simulink model "sensorFusionWithControlTB66StatePos"  (R2024a)
settings: Solver=FixedStepAuto  StartTime=0.0  StopTime=inf  FixedStep=controlRate  RelTol=1e-3
InitFcn:
  | modelParamsDD = Simulink.data.dictionary.open('modelConfigData.sldd');
  | sectModel = getSection(modelParamsDD,'Design Data');
  | controlRateTemp = getValue(getEntry(sectModel,'controlRate'));
  | 
  | measRate = controlRateTemp;
  | angleEstRate = measRate;
  | stateEstRate = measRate;
  | 
  | 
  | % Complementary filter
  | fc = 5; %Hz
  | tau = 1/(2*pi*fc);
  | alpha = tau/(tau+controlRateTemp);
  | 
  | % Control params
  | tiltSetPoint = 1; % degree
  | 
  | % Tilt angle PID
  | Tw = 1;
  | Kp = 17;
  | Ki = 4; %
  | Kd = 0;
  | 
  | % Velocity angle PID
  | Tw_vel = 1;
  | Kp_vel = 17;
  | Ki_vel = 4;
  | Kd_vel = 0;
  | 
  | % Position angle PID
  | targetPosition = 0.1;
  | Tw_pos = 1;
  | Kp_pos = 17;
  | Ki_pos = 4;
  | Kd_pos = 0;
  | 
  | clear controlRateTemp
  | 
  | motorParamsDD = Simulink.data.dictionary.open('motorParametersData.sldd');
  | robotParamsDD = Simulink.data.dictionary.open('robotModelData.sldd');
  | controlParamsDD = Simulink.data.dictionary.open('controlVariablesData.sldd');
  | sectMotor = getSection(motorParamsDD,'Design Data');
  | sectRobot = getSection(robotParamsDD,'Design Data');
  | sectControl = getSection(controlParamsDD,'Design Data');
  | 
  | % Physical Parameters
  | M = getValue(getEntry(sectRobot,'massOfCart'));    % mass of cart
  | m = getValue(getEntry(sectRobot,'massOfPendulum'));    % mass of pendulum
  | L = getValue(getEntry(sectRobot,'lengthToPendulumCenterOfMass'));    % length to pendulum center of mass
  | g = 9.81;   % gravity
  | I = getValue(getEntry(sectRobot,'inertiaOfPendulum'));  % inertia of pendulum
  | r = getValue(getEntry(sectRobot,'wheelRadius'));   % 5 cm wheel radius
  | 
  | % Servo motor state: i, omega
  | Rm = getValue(getEntry(sectMotor,'armatureResistance')); % motor resistance
  | Lm = getValue(getEntry(sectMotor,'armatureInductance')); % motor coil inductance
  | Km = getValue(getEntry(sectMotor,'motorTorqueConstantKm')); % motor torque constant
  | Kb = getValue(getEntry(sectMotor,'backEMFConstantKb')); % motor electrical consant
  | Kf = getValue(getEntry(sectMotor,'viscousFriction')); % viscous friction
  | J = getValue(getEntry(sectMotor,'motorInertia'));  % inertia of rotor
  | 
  | Q_aug_lqr = getValue(getEntry(sectControl,'Q_aug_lqr'));
  | R_aug_lqr = getValue(getEntry(sectControl,'R_aug_lqr'));
  | 
  | % States are x, dx/dt, phi, dphi/dt
  | % Outputs are x position and tilt angle
  | 
  | % Linearized state-space model of inverted pendulum
  | I_tot = m*L^2+I;
  | p = m^2*L^2 - I_tot*(M+m);
  | A_pend = [0 1 0 0;
  |           0 0 (m^2 * g * L^2)/p 0;
  |           0 0 0 1;
  |           0 0 -(M+m)/(m*L)*m^2*L^2*g/p 0];
  | 
  | B_pend = [0; -I_tot/p; 0; 1/(m*L)*(1+(M+m)*I_tot/p)];
  | 
  | C_pend = [1 0 0 0;
  |           0 0 1 0];
  | D_pend = zeros(2,1);
  | 
  | % Discretize System - for the augmented system
  | sysd = c2d(ss(A_pend, B_pend, C_pend, D_pend), measRate);
  | Ad_pend = single(sysd.A);
  | Bd_pend = single(sysd.B);
  | Cd_pend = single(sysd.C);
  | Dd_pend = single(sysd.D);
  | 
  | % State-space model: output is torque = Km * i
  | A_motor = [-Rm/L,   -Kb/Lm;
  |             Km/J, -Kf/J];
  | B_motor = [1/Lm;
  |            0];
  | C_motor = [Km*(1/r), 0];  % Output is torque = Km * i
  | D_motor = 0;
  | 
  | % Augment System: Force = torque / r
  | % States are x, dx/dt, phi, dphi/dt, i, w
  | % Outputs are x position and tilt angle
  | 
  | A_aug = [A_pend, B_pend*C_motor;
  |          zeros(2,4), A_motor];
  | 
  | B_aug = [B_pend*D_motor; B_motor];
  | 
  | C_aug = [C_pend, D_pend*C_motor];
  | n_aug = size(A_aug,1);
  | 
  | 
  | % Discretize System - for the augmented system
  | sysd = c2d(ss(A_aug, B_aug, C_aug, 0), measRate);
  | Ad_aug = single(sysd.A);
  | Bd_aug = single(sysd.B);
  | Cd_aug = single(sysd.C);
  | 
  | clear J Kt M m l g I r Q_lqr_temp R_lqr_temp dt
  | clear Rm Lm Km Kb Kf J
  | clear motorParamsDD robotParamsDD controlParamsDD modelParamsDD sectMotor sectRobot sectControl sectModel sysd
  | 
  | % LQR Controller matrices (moved here from SLDD to be tuned)
  | Q_aug_lqr_temp = [0.1 0 0 0 0 0;0 0.1 0 0 0 0;0 0 10 0 0 0;0 0 0 50 0 0;0 0 0 0 0.1 0;0 0 0 0 0 0.1];
  | R_aug_lqr_temp = 30;
  | 
  | % LQR Controller - for the augmented system
  | [K_aug_lqr, ~, ~] = dlqr(Ad_aug, Bd_aug, Q_aug_lqr, R_aug_lqr);
  | K_aug_lqr = single(K_aug_lqr);
undefined symbols (not defined in the file or in its folder): accelToUnit, controlRate, gyroToUnit, MaxMotorVoltage, posControlRate
libraries: stm32blockslib x2, stm32f7xxblockslib x2, stm32f4xxblockslib x1
settings Model: DataDictionary=globalData.sldd  VariantConfigurationObject=RobotVariantConfig  STM32="{\"PWMOutput\":[{\"ID\":\"sensorFusionWithControlTB66State:205\"},{\"ID\":\"sensorFusionWithControlTB66State:189\"},{\"ID\":\"sensorFusionWithControlTB66StatePos:2012\"},{\"ID\":\"sensorFusionWithControlTB66StatePos:2013\"}],\"DigitalPortWrite\":[{\"ID\":\"sensorFusionWithControlTB66State:1189\"},{\"ID\":\"sensorFusionWithControlTB66State:1225:7\"},{\"ID\":\"sensorFusionWithControlTB66State:1225:8\"},{\"ID\":\"sensorFusionWithControlTB66State:1225:9\"},{\"ID\":\"sensorFusionWithControlTB66State:1225:10\"},{\"ID\":\"sensorFusionWithControlTB66StatePos:1992\"},{\"ID\":\"sensorFusionWithControlTB66StatePos:2051:7\"},{\"ID\":\"sensorFusionWithControlTB66StatePos:2051:8\"},{\"ID\":\"sensorFusionWithControlTB66StatePos:2051:9\"},{\"ID\":\"sensorFusionWithControlTB66StatePos:2051:10\"}],\"EncoderBlock\":[{\"ID\":\"sensorFusionWithControlTB66State:1254\"},{\"ID\":\"sensorFusionWithControlTB66State:1257\"},{\"ID\":\"sensorFusionWithControlTB66StatePos:1993\"},{\"ID\":\"sensorFusionWithControlTB66StatePos:1994\"}],\"I2CControllerRead\":[{\"ID\":\"sensorFusionWithControlTB66State:1237:7\"},{\"ID\":\"sensorFusionWithControlTB66State:1237:18\"},{\"ID\":\"sensorFusionWithControlTB66State:1237:19\"},{\"ID\":\"sensorFusionWithControlTB66State:1237:20\"},{\"ID\":\"sensorFusionWithControlTB66State:1238:7\"},{\"ID\":\"sensorFusionWithControlTB66State:1238:15\"},{\"ID\":\"sensorFusionWithControlTB66State:1238:16\"},{\"ID\":\"sensorFusionWithControlTB66State:1238:17\"},{\"ID\":\"sensorFusionWithControlTB66StatePos:1237:18\"},{\"ID\":\"sensorFusionWithControlTB66StatePos:1237:19\"},{\"ID\":\"sensorFusionWithControlTB66StatePos:1237:20\"},{\"ID\":\"sensorFusionWithControlTB66StatePos:1238:7\"},{\"ID\":\"sensorFusionWithControlTB66StatePos:1238:15\"},{\"ID\":\"sensorFusionWithControlTB66StatePos:1238:16\"},{\"ID\":\"sensorFusionWithControlTB66StatePos:1238:17\"},{\"ID\":\"sensorFusionWithControlTB66StatePos:2053:7\"},{\"ID\":\"sensorFusionWithControlTB66StatePos:2053:18\"},{\"ID\":\"sensorFusionWithControlTB66StatePos:2053:19\"},{\"ID\":\"sensorFusionWithControlTB66StatePos:2053:20\"},{\"ID\":\"sensorFusionWithControlTB66StatePos:2054:7\"},{\"ID\":\"sensorFusionWithControlTB66StatePos:2054:15\"},{\"ID\":\"sensorFusionWithControlTB66StatePos:2054:16\"},{\"ID\":\"sensorFusionWithControlTB66StatePos:2054:17\"}],\"I2CControllerWrite\":[{\"ID\":\"sensorFusionWithControlTB66State:1237:21\"},{\"ID\":\"sensorFusionWithControlTB66State:1237:22\"},{\"ID\":\"sensorFusionWithControlTB66State:1237:23\"},{\"ID\":\"sensorFusionWithControlTB66State:1238:18\"},{\"ID\":\"sensorFusionWithControlTB66State:1238:19\"},{\"ID\":\"sensorFusionWithControlTB66State:1238:20\"},{\"ID\":\"sensorFusionWithControlTB66StatePos:1237:21\"},{\"ID\":\"sensorFusionWithControlTB66StatePos:1237:22\"},{\"ID\":\"sensorFusionWithControlTB66StatePos:1237:23\"},{\"ID\":\"sensorFusionWithControlTB66StatePos:1238:18\"},{\"ID\":\"sensorFusionWithControlTB66StatePos:1238:19\"},{\"ID\":\"sensorFusionWithControlTB66StatePos:1238:20\"},{\"ID\":\"sensorFusionWithControlTB66StatePos:2053:21\"},{\"ID\":\"sensorFusionWithControlTB66StatePos:2053:22\"},{\"ID\":\"sensorFusionWithControlTB66StatePos:2053:23\"},{\"ID\":\"sensorFusionWithControlTB66StatePos:2054:18\"},{\"ID\":\"sensorFusionWithControlTB66StatePos:2054:19\"},{\"ID\":\"sensorFusionWithControlTB66StatePos:2054:20\"}]}"  SimulationMode=external  Creator=Peter  LastModifiedBy=Peter
settings OptimizationCC: OptimizeBlockIOStorage=off  BufferReuse=off  ReuseModelBlockBuffer=off  GlobalBufferReuse=off  ExpressionFolding=off  EnableMemcpy=off  PassReuseOutputArgsAs=Individual arguments  LocalBlockOutputs=off  ZeroExternalMemoryAtStartup=off  ZeroInternalMemoryAtStartup=off  MaxStackSize=64  OptimizeDataStoreBuffers=off  BusAssignmentInplaceUpdate=off  OptimizationLevel=level0  OptimizationCustomize=off  EfficientTunableParamExpr=on
settings DebuggingCC: ParameterTunabilityLossMsg=error
settings HardwareCC: ProdBitPerPointer=32  ProdBitPerSizeT=32  ProdBitPerPtrDiffT=32  ProdLargestAtomicInteger=Long  ProdLargestAtomicFloat=Double  ProdWordSize=32  ProdLongLongMode=on  ProdHWDeviceType=ARM Compatible->ARM Cortex-M
settings SFSimCC: MATLABDynamicMemAlloc=off
settings RTWCC: Description=Embedded Coder  SystemTargetFile=ert.tlc  HardwareBoard=STM32F7xx Based (Single precision FPU)  GenCodeOnly=on  TemplateMakefile=ert_default_tmf  Toolchain=GNU Tools for ARM Embedded Processors
settings CodeAppCC: GenerateComments=off  IgnoreCustomStorageClasses=off  OperatorAnnotations=on  SimulinkDataObjDesc=on  SFDataObjDesc=on  SimulinkBlockComments=off
settings ERTTargetCC: TargetLangStandard=C99 (ISO)  CodeReplacementLibrary=ARM Cortex-M  SupportComplex=off  ExtMode=on  ExtModeTransport=3  ExtModeStaticAlloc=on  ExtModeStaticAllocSize=2048  ExtModeMexFile=ext_xcp  ExtModeMexArgs=1 'COM11' 115200  ExtModeIntrfLevel=Level2 - Open

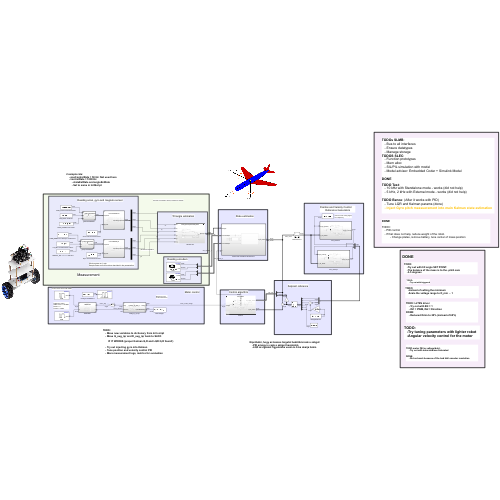
[thumbnail: Simulink's stored preview of the top-level diagram]
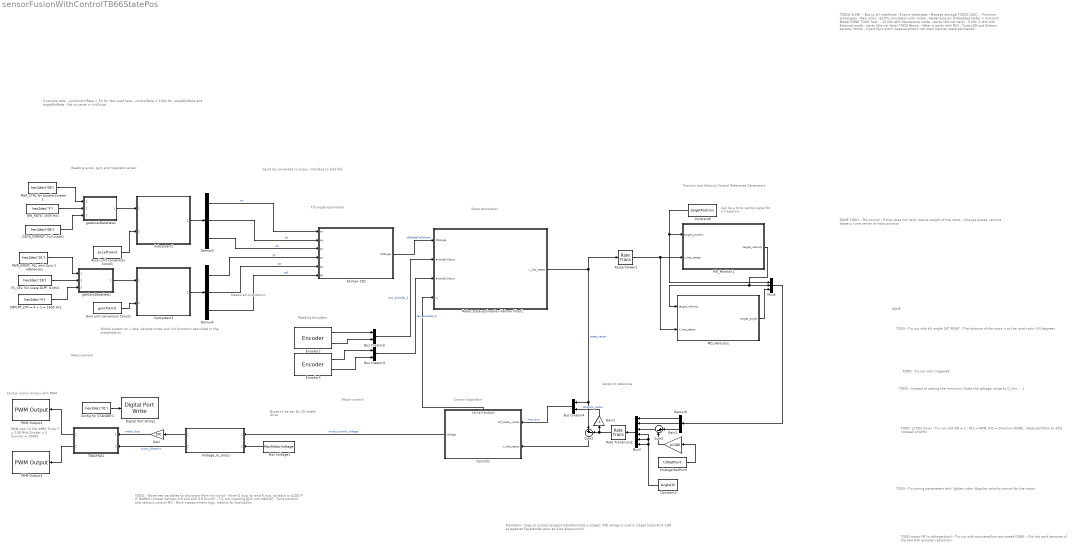
== system sensorFusionWithControlTB66StatePos ==
  note: Control algorithm
  note: Control motor dirvers with PWM
  note: TODO:
      | -Try out with tilt angle SET POINT.
      | -The balance of the mass is to the -pitch axis
      | -3-5 degrees
  note: TODO motor FB (w voltage/duty)
      | - Try out with saturated/non saturated
      |
      | DONE:
      | - Did not work because of the bad Hall encoder resolution
  note: Reading accel, gyro and megneto sensor
  note: Measured orientation
  note: 2 sample rate:
      | - posControlRate = 50 Hz: Not used here
      | - controlRate = 1000 Hz
      | - stateEstRate and angleEstRate
      | - Set to same in InitScript
  note: PWM with 10 kHz
      | APB2 Timer f = 108 MHz
      | Divider = 0
      | Counter = 10800
  note: Measurement
  note: Motor control
  note: Whole system on 1 rate.
      | Sample times and init functions described in the presentation.
  note: Buses to be set
      | for 2D wheel drive
  note: State estimation
  note: Setpoint reference
  note: Tilt angle estimation
  note: TODO:
      | -Try tuning parameters with lighter robot
      | -Angular velocity control for the motor
  note: Reading encoders
  note: Could be converted to buses, interface to sldd file
  note: TODO:
      | -Try out with triggered
  note: TODO: L279N driver
      | - Try out with EN = 1
      | - IN1 = PWM, IN2 = Direction
      | DONE:
      | - Reduced Dmin to 20% (instead of 60%)
  note: DONE
  note: TODO:
      | -Instead of setting the minimum
      | -Scale the voltage range to D_min ... 1
  note: DONE
      |
      | TODO:
      | - PID control
      | - If that does not help, reduce weight of the robot.
      | - Change plates, remove battery, tune center of mass position
  note: TODOs SLMB :
      | - Bus to all interfaces
      | - Ensure datatypes
      | - Manage storage
      | TODOS SLEC :
      | - Function prototypes
      | - Mem alloc
      | - SIL/PIL simulation with model
      | - Model advisor: Embedded Coder + Simulink Model
      |
      | DONE
      |
      | TODO Test :
      | - 10 kHz with Standalone mode - works (did not help)
      | - 5 kHz, 2 kHz with External mode - works (did not help)
      |
      | TODO Bence : (After it works with PID)
      | - Tune LQR and Kalman params (done)
      | - Inject Gyro pitch measuerement into main Kalman state estimation
  note: TODO:
      | - Move new variables to dictionary from Init script
      | - Move Q_aug_lqr and R_aug_lqr back to SLDD
      |
      | IF IT WORKS (proper Kalman Q,R and LQR Q,R found!)
      |
      | - Try out injecting gyro into Kalman
      | - Tune position and velocity control PID
      | - More measurement logs, metrics for evaluation
  note: Can be a time varing signal
      | for a trajectory
  note: Kipróbálni, hogy az összes targetot bekötöm/csak a szöget:
      | -PID amúgy is csak a szöget használná
      | -LQR az egészet figyelembe veszi és 0-ba akarja húzni.
  note: Position and Velocity Control
      | Reference Generators
  Accel unit conversion Const1 : Constant  Value=accelToUnit  OutDataTypeStr=single
  BW_RATE: 1600 Hz1 : Constant  Value=hex2dec('F')  OutDataTypeStr=uint8
  Bus Creator2 : BusCreator  Inputs=2
  Bus Creator3 : BusCreator  Inputs=2
  Bus Creator4 : BusCreator  Inputs=2
  Config for STANDBY1 : Constant  Value=hex2dec('01')  OutDataTypeStr=uint8
  Constant2 : Constant  Value=single(0)
  Constant6 : Constant  Value=targetPosition  OutDataTypeStr=single
  Control1 : Subsystem  Variant=on  VariantChoicesEnumeration=controlEnumState  VariantControlVariable=controlAlgStateCtrl  VariantControl=Subsystem2  VariantActivationTime=inherit from Simulink.VariantControl
      settings: PortSchema="{\"entries\":[{\"content\":{\"sides\":[{\"content\":{\"connectorIds\":[\"In1\",\"In2\"]},\"type\":\"ConnectorPlacement.EquallySpacedRectSide\",\"uuid\":\"f699f757-4844-4aff-9ceb-41d5b2044f89\"},{\"content\":{\"connectorIds\":[\"Out1\"],\"side\":\"RIGHT\"},\"type\":\"ConnectorPlacement.EquallySpacedRectSide\",\"uuid\":\"5d4ff76b-5e14-4a3a-b7d6-9f05c394657c\"},{\"content\":{\"connectorIds\":[\"Out2\"],\"side\":\"TOP\"},\"type\":\"ConnectorPlacement.EquallySpacedRectSide\",\"uuid\":\"774b8687-b42a-4b88-b210-7c8eb4b61568\"}]},\"type\":\"ConnectorPlacement.EquallySpacedConnector\",\"uuid\":\"f6913896-c1bf-44b7-bb24-894f4bed7d15\"}],\"packageUris\":[\"http://schema.mathworks.com/mf0/Connector/R2020b\"],\"version\":\"1.0\"}"
  DATA_FORMAT: Full scale1 : Constant  Value=hex2dec('0B')  OutDataTypeStr=uint8
  Demux3 : Demux  Outputs=3
  Demux4 : Demux  Outputs=3
  Demux6 : Demux  Outputs=3
  Digital Port Write1 : stm32f4xxblockslib/Digital Port Write  PortName=GPIOF  PinNumber=[13]  ReadOperation=off  IOAsArray=off  EnableSimPort=off  hoistedMaskSrc=ECSoC/ECSimCodegen/Digital Port Write
      settings: LibrarySourceBlock=stm32f7xxblockslib/Digital Port Write
  Encoder2 : stm32blockslib/Encoder  TimerModule=TIM1  EnableResetInput=off  OutputDirection=on  SampleTime=angleEstRate
      settings: LibrarySourceBlock=stm32f7xxblockslib/Encoder
  Encoder3 : stm32blockslib/Encoder  TimerModule=TIM3  EnableResetInput=off  OutputDirection=on  SampleTime=angleEstRate
      settings: LibrarySourceBlock=stm32f7xxblockslib/Encoder
  FS_SEL: full scale DLPF: 8 kHz1 : Constant  Value=hex2dec('18')  OutDataTypeStr=uint8
  FasterSlower1 : RateTransition
  Gain : Gain  Gain=100
  Gain1 : Gain  Gain=pi/180  ParamDataTypeStr=single
  Gain2 : Gain  Gain=-1
  Gyro unit conversion Const1 : Constant  Value=gyroToUnit  OutDataTypeStr=single
  Kalman 2D1 : Subsystem  Variant=on  VariantChoicesEnumeration=tiltEnum  VariantControlVariable=tiltEstCtrl  VariantControl=Kalman 2D  VariantActivationTime=inherit from Simulink.VariantControl
  Max Voltage1 : Constant  Value=MaxMotorVoltage  OutDataTypeStr=single
  Mux2 : Mux  Inputs=6
  Mux4 : Mux  Inputs=3
  PID_Position1 : Subsystem  TreatAsAtomicUnit=on  SystemSampleTime=posControlRate
  PID_Velocity1 : Subsystem  TreatAsAtomicUnit=on  SystemSampleTime=posControlRate
  PWM Output2 : stm32f7xxblockslib/PWM Output  TimerModule=TIM8  DutycycleUnits=Percentage  EnableChannel1=off  EnableChannel2=off  EnableChannel3=on  EnableChannel4=off  EnableChannel5=off  EnableChannel6=off  EnableCounterInput=off  EnableMainOutputInput=off  EnableFrequencyInput=off  SetRCAfterCE=off  OutputDirection=off  OutputMainOutputEnableStatus=off  SampleTime=0.1  EnableSimPort=off  EnableUpdateEvent=off  EnableCaptureCompare1Event=off  EnableCaptureCompare2Event=off  EnableCaptureCompare3Event=off  EnableCaptureCompare4Event=off  EnableTriggerEvent=off  EnableBreakEvent=off  EnableBreakEvent2=off  ProcessorFamily=STM32F7  hoistedMaskSrc=ECSoC/ECSimCodegen/PWM Output
  PWM Output3 : stm32f7xxblockslib/PWM Output  TimerModule=TIM8  DutycycleUnits=Percentage  EnableChannel1=off  EnableChannel2=off  EnableChannel3=off  EnableChannel4=on  EnableChannel5=off  EnableChannel6=off  EnableCounterInput=off  EnableMainOutputInput=off  EnableFrequencyInput=off  SetRCAfterCE=off  OutputDirection=off  OutputMainOutputEnableStatus=off  SampleTime=0.1  EnableSimPort=off  EnableUpdateEvent=off  EnableCaptureCompare1Event=off  EnableCaptureCompare2Event=off  EnableCaptureCompare3Event=off  EnableCaptureCompare4Event=off  EnableTriggerEvent=off  EnableBreakEvent=off  EnableBreakEvent2=off  ProcessorFamily=STM32F7  hoistedMaskSrc=ECSoC/ECSimCodegen/PWM Output
  PWR_CTRL for Accelerometer1 : Constant  Value=hex2dec('08')  OutDataTypeStr=uint8
  PWR_MGMT: PLL with Gyro X reference1 : Constant  Value=hex2dec('01')  OutDataTypeStr=uint8
  Rate Transition2 : RateTransition
  Robot state estimation Kalman filter1 : Subsystem  TreatAsAtomicUnit=on  SystemSampleTime=stateEstRate
  SMPLRT_DIV = 4 + 1 = 1600 Hz1 : Constant  Value=hex2dec('4')  OutDataTypeStr=uint8
  Subsystem2 : Subsystem  TreatAsAtomicUnit=on  SystemSampleTime=angleEstRate  ReferencedSubsystem=convertRawAccel
  Subsystem3 : Subsystem  TreatAsAtomicUnit=on  SystemSampleTime=angleEstRate  ReferencedSubsystem=convertRawGyro
  Sum2 : Sum  Inputs=|+-
  Sum5 : Sum  Inputs=|+-
  TB66FNG1 : Subsystem  TreatAsAtomicUnit=on  SystemSampleTime=controlRate  ReferencedSubsystem=TB66FNG
  Voltage_to_duty1 : Subsystem  TreatAsAtomicUnit=on  SystemSampleTime=controlRate  ReferencedSubsystem=Voltage_to_duty_1
  getAccelDataNew1 : Subsystem  TreatAsAtomicUnit=on  ReferencedSubsystem=getAccelDataNew
  getGyroDataNew1 : Subsystem  TreatAsAtomicUnit=on  ReferencedSubsystem=getGyroDataNew
  tiltAngelSetPoint : Constant  Value=tiltSetPoint  OutDataTypeStr=single
  wires:
  Control1/2(kalmanFeedback) -> Robot state estimation Kalman filter1/4(u)
  Encoder2/1 -> Bus Creator2/1
  Bus Creator4/1 -> Control1/1(ref_state_vector)  "mpc_bus"
  Subsystem3/1 -> Demux4/1
  Encoder3/2 -> Bus Creator3/2
  Bus Creator3/1 -> Robot state estimation Kalman filter1/3(encoder2Input)  "raw_encoder_2"
  Bus Creator2/1 -> Robot state estimation Kalman filter1/2(encoder1Input)  "raw_encoder_1"
  Encoder3/1 -> Bus Creator3/1
  SMPLRT_DIV = 4 + 1 = 1600 Hz1/1 -> getGyroDataNew1/3
  Gain/1 -> TB66FNG1/1  "motor_duty"
  Gain2/1 -> Bus Creator4/2  "setpoint_vector"
  Encoder2/2 -> Bus Creator2/2
  Demux3/1 -> Kalman 2D1/1(ax)  "ax"
  PWR_CTRL for Accelerometer1/1 -> getAccelDataNew1/1
  Gain1/1 -> Sum5/2
  TB66FNG1/1 -> PWM Output2/1
  Subsystem2/1 -> Demux3/1
  TB66FNG1/2 -> PWM Output3/1
  tiltAngelSetPoint/1 -> Gain1/1
  Mux2/1 -> Rate Transition2/1
  Accel unit conversion Const1/1 -> Subsystem2/2
  Voltage_to_duty1/2 -> TB66FNG1/2  "motor_direction"
  getAccelDataNew1/1 -> Subsystem2/1
  FS_SEL: full scale DLPF: 8 kHz1/1 -> getGyroDataNew1/2
  Kalman 2D1/1(tiltAngle) -> Robot state estimation Kalman filter1/1(tiltAngle)  "tiltAngleToKalman"
  DATA_FORMAT: Full scale1/1 -> getAccelDataNew1/3
  Gyro unit conversion Const1/1 -> Subsystem3/2
  Sum2/1 -> Control1/2(x_hat_states)
  BW_RATE: 1600 Hz1/1 -> getAccelDataNew1/2
  Demux4/2 -> Kalman 2D1/5(gy)  "gy"
  Max Voltage1/1 -> Voltage_to_duty1/2
  Control1/1(voltage) -> Voltage_to_duty1/1  "motor_control_voltage"
  PWR_MGMT: PLL with Gyro X reference1/1 -> getGyroDataNew1/1
  Demux3/2 -> Kalman 2D1/2(ay)  "ay"
  Voltage_to_duty1/1 -> Gain/1
  getGyroDataNew1/1 -> Subsystem3/1
  Demux4/1 -> Kalman 2D1/4(gx)  "gx"
  Config for STANDBY1/1 -> Digital Port Write1/1
  Demux4/3 -> Kalman 2D1/6(gz)  "gzf"
  Demux3/3 -> Kalman 2D1/3(az)  "az"
  Mux4/1 -> Demux6/1
  PID_Velocity1/1(target_angle) -> Mux4/3
  PID_Position1/1(target_velocity) -> Mux4/2, PID_Velocity1/1(target_velocity)
  Constant6/1 -> Mux4/1, PID_Position1/1(target_position)
  FasterSlower1/1 -> PID_Velocity1/2(x_hat_states), PID_Position1/2(x_hat_states)
  Robot state estimation Kalman filter1/1(x_hat_states) -> Bus Creator4/1, Sum2/1, FasterSlower1/1  "state_vector"
  Constant2/1 -> Mux2/4, Mux2/5, Mux2/6
  Sum5/1 -> Mux2/3
  Rate Transition2/1 -> Gain2/1, Sum2/2
  Demux6/3 -> Sum5/1
  Demux6/2 -> Mux2/2
  Demux6/1 -> Mux2/1

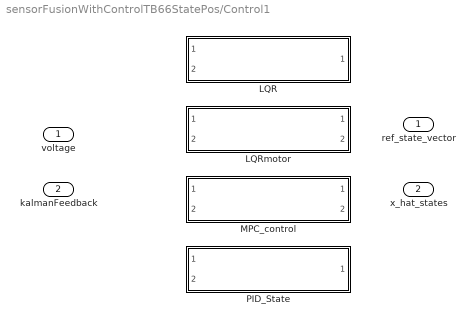
== system sensorFusionWithControlTB66StatePos/Control1 ==
  ref_state_vector : Inport
  x_hat_states : Inport  Port=2  OutDataTypeStr=single
  LQR : Subsystem  SystemSampleTime=controlRate  VariantControl=controlAlgStateCtrl == controlEnumState.LQR  ReferencedSubsystem=LQR
  LQRmotor : Subsystem  SystemSampleTime=controlRate  VariantControl=controlAlgStateCtrl == controlEnumState.LQRmotor  ReferencedSubsystem=LQRmotor
  MPC_control : Subsystem  VariantControl=controlAlgStateCtrl == controlEnumState.MPC_control  ReferencedSubsystem=MPC_control
  PID_State : Subsystem  VariantControl=controlAlgStateCtrl == controlEnumState.PID_State  ReferencedSubsystem=PID_State
  voltage : Outport  OutDataTypeStr=single
  kalmanFeedback : Outport  Port=2  OutDataTypeStr=single

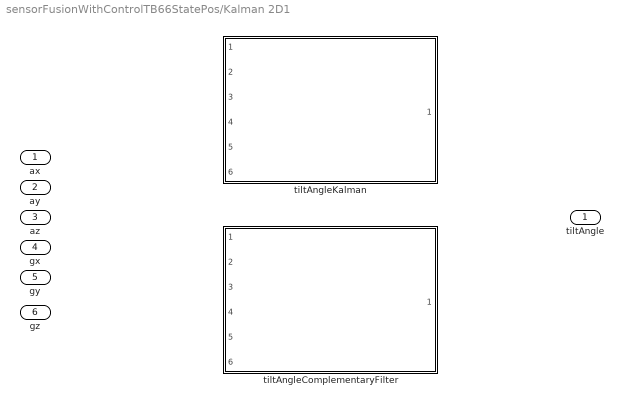
== system sensorFusionWithControlTB66StatePos/Kalman 2D1 ==
  ax : Inport
  ay : Inport  Port=2
  az : Inport  Port=3
  gx : Inport  Port=4
  gy : Inport  Port=5
  gz : Inport  Port=6
  tiltAngleComplementaryFilter : Subsystem  TreatAsAtomicUnit=on  SystemSampleTime=controlRate  VariantControl=tiltEstCtrl == tiltEnum.tiltAngleComplementaryFilter  ReferencedSubsystem=tiltAngleComplementaryFilter
  tiltAngleKalman : Subsystem  TreatAsAtomicUnit=on  SystemSampleTime=angleEstRate  VariantControl=tiltEstCtrl == tiltEnum.tiltAngleKalman  ReferencedSubsystem=tiltAngleKalman
  tiltAngle : Outport

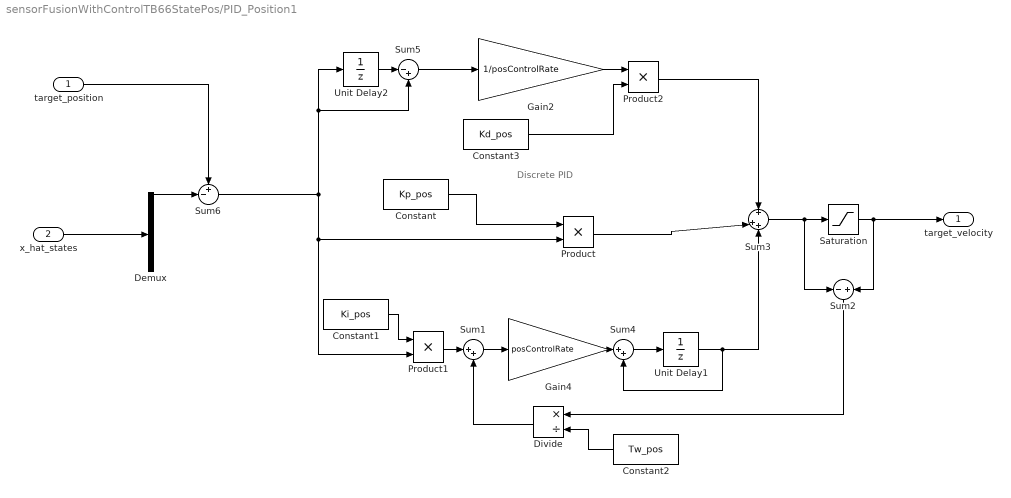
== system sensorFusionWithControlTB66StatePos/PID_Position1 ==
  note: Discrete PID
  target_position : Inport
  x_hat_states : Inport  Port=2
  Constant : Constant  Value=Kp_pos  OutDataTypeStr=single
  Constant1 : Constant  Value=Ki_pos  OutDataTypeStr=single
  Constant2 : Constant  Value=Tw_pos  OutDataTypeStr=single
  Constant3 : Constant  Value=Kd_pos  OutDataTypeStr=single
  Demux : Demux  Outputs=6
  Divide : Product  Inputs=*/
  Gain2 : Gain  Gain=1/posControlRate  ParamDataTypeStr=single
  Gain4 : Gain  Gain=posControlRate  ParamDataTypeStr=single
  Product : Product
  Product1 : Product
  Product2 : Product
  Saturation : Saturate  UpperLimit=12  LowerLimit=-12  OutDataTypeStr=single
  Sum1 : Sum  Inputs=|++
  Sum2 : Sum  Inputs=-|+
  Sum3 : Sum  Inputs=+|++
  Sum4 : Sum  Inputs=|++
  Sum5 : Sum  Inputs=|-+
  Sum6 : Sum  Inputs=+-|
  Unit Delay1 : UnitDelay  SampleTime=-1  HasFrameUpgradeWarning=on
  Unit Delay2 : UnitDelay  SampleTime=-1  HasFrameUpgradeWarning=on
  target_velocity : Outport
  wires:
  Constant/1 -> Product/1
  Constant2/1 -> Divide/2
  Unit Delay2/1 -> Sum5/1
  Sum6/1 -> Product1/2, Product/2, Unit Delay2/1, Sum5/2
  Gain4/1 -> Sum4/1
  Sum3/1 -> Sum2/1, Saturation/1
  x_hat_states/1 -> Demux/1
  Sum4/1 -> Unit Delay1/1
  Constant1/1 -> Product1/1
  Sum5/1 -> Gain2/1
  Sum1/1 -> Gain4/1
  Gain2/1 -> Product2/1
  Sum2/1 -> Divide/1
  Divide/1 -> Sum1/2
  Product/1 -> Sum3/2
  Product2/1 -> Sum3/1
  Saturation/1 -> target_velocity/1, Sum2/2
  Product1/1 -> Sum1/1
  Constant3/1 -> Product2/2
  Unit Delay1/1 -> Sum3/3, Sum4/2
  Demux/1 -> Sum6/2
  target_position/1 -> Sum6/1

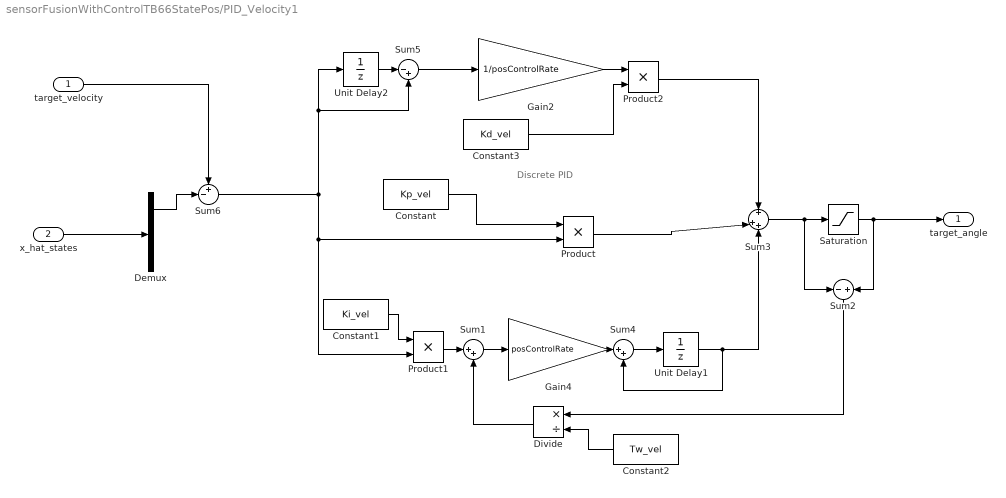
== system sensorFusionWithControlTB66StatePos/PID_Velocity1 ==
  note: Discrete PID
  target_velocity : Inport
  x_hat_states : Inport  Port=2
  Constant : Constant  Value=Kp_vel  OutDataTypeStr=single
  Constant1 : Constant  Value=Ki_vel  OutDataTypeStr=single
  Constant2 : Constant  Value=Tw_vel  OutDataTypeStr=single
  Constant3 : Constant  Value=Kd_vel  OutDataTypeStr=single
  Demux : Demux  Outputs=6
  Divide : Product  Inputs=*/
  Gain2 : Gain  Gain=1/posControlRate  ParamDataTypeStr=single
  Gain4 : Gain  Gain=posControlRate  ParamDataTypeStr=single
  Product : Product
  Product1 : Product
  Product2 : Product
  Saturation : Saturate  UpperLimit=12  LowerLimit=-12  OutDataTypeStr=single
  Sum1 : Sum  Inputs=|++
  Sum2 : Sum  Inputs=-|+
  Sum3 : Sum  Inputs=+|++
  Sum4 : Sum  Inputs=|++
  Sum5 : Sum  Inputs=|-+
  Sum6 : Sum  Inputs=+-|
  Unit Delay1 : UnitDelay  SampleTime=-1  HasFrameUpgradeWarning=on
  Unit Delay2 : UnitDelay  SampleTime=-1  HasFrameUpgradeWarning=on
  target_angle : Outport
  wires:
  target_velocity/1 -> Sum6/1
  Demux/2 -> Sum6/2
  Unit Delay1/1 -> Sum4/2, Sum3/3
  Constant3/1 -> Product2/2
  Product1/1 -> Sum1/1
  Saturation/1 -> Sum2/2, target_angle/1
  Product2/1 -> Sum3/1
  Product/1 -> Sum3/2
  Divide/1 -> Sum1/2
  Sum2/1 -> Divide/1
  Gain2/1 -> Product2/1
  Sum1/1 -> Gain4/1
  Sum5/1 -> Gain2/1
  Constant1/1 -> Product1/1
  Sum4/1 -> Unit Delay1/1
  x_hat_states/1 -> Demux/1
  Sum3/1 -> Saturation/1, Sum2/1
  Gain4/1 -> Sum4/1
  Sum6/1 -> Sum5/2, Unit Delay2/1, Product/2, Product1/2
  Unit Delay2/1 -> Sum5/1
  Constant2/1 -> Divide/2
  Constant/1 -> Product/1

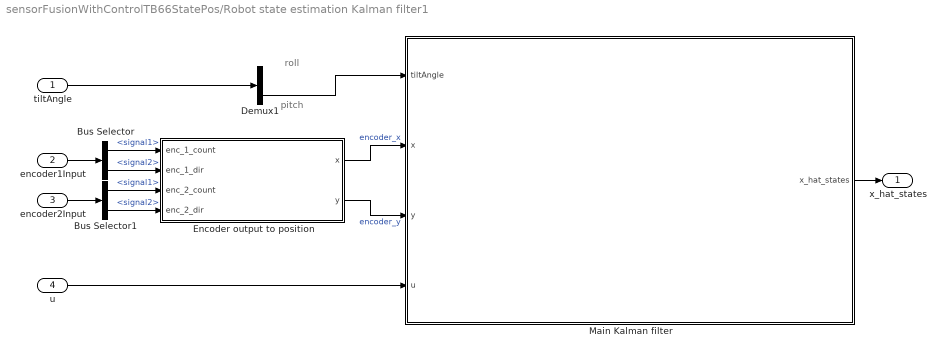
== system sensorFusionWithControlTB66StatePos/Robot state estimation Kalman filter1 ==
  note: pitch
  note: roll
  tiltAngle : Inport
  encoder1Input : Inport  Port=2
  encoder2Input : Inport  Port=3
  u : Inport  Port=4
  Bus Selector : BusSelector  OutputSignals=signal1,signal2
  Bus Selector1 : BusSelector  OutputSignals=signal1,signal2
  Demux1 : Demux  Outputs=2
  Encoder output to position : Subsystem  Variant=on  VariantChoicesEnumeration=encoderDimEnum  VariantControlVariable=encoderDimCtrl  VariantControl=Encoder output to position  VariantActivationTime=inherit from Simulink.VariantControl
  Main Kalman filter : Subsystem  Variant=on  VariantChoicesEnumeration=mainStateEnum  VariantControlVariable=mainStateEstCtrl  VariantControl=Subsystem1  VariantActivationTime=inherit from Simulink.VariantControl
  x_hat_states : Outport  OutDataTypeStr=single
  wires:
  tiltAngle/1 -> Demux1/1
  Main Kalman filter/1(x_hat_states) -> x_hat_states/1
  Bus Selector/1 -> Encoder output to position/1(enc_1_count)  "<signal1>"
  Bus Selector/2 -> Encoder output to position/2(enc_1_dir)  "<signal2>"
  Encoder output to position/1(x) -> Main Kalman filter/2(x)  "encoder_x"
  Encoder output to position/2(y) -> Main Kalman filter/3(y)  "encoder_y"
  u/1 -> Main Kalman filter/4(u)
  Demux1/2 -> Main Kalman filter/1(tiltAngle)
  encoder1Input/1 -> Bus Selector/1
  encoder2Input/1 -> Bus Selector1/1
  Bus Selector1/1 -> Encoder output to position/3(enc_2_count)  "<signal1>"
  Bus Selector1/2 -> Encoder output to position/4(enc_2_dir)  "<signal2>"

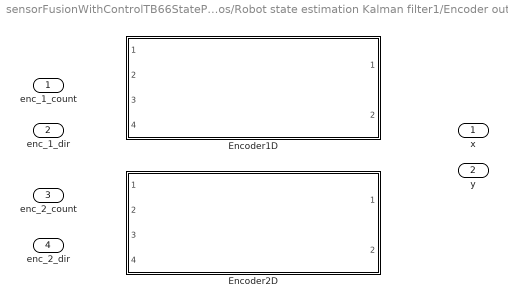
== system sensorFusionWithControlTB66StatePos/Robot state estimation Kalman filter1/Encoder output to position ==
  enc_1_count : Inport
  enc_1_dir : Inport  Port=2
  enc_2_count : Inport  Port=3
  enc_2_dir : Inport  Port=4
  Encoder1D : Subsystem  VariantControl=encoderDimCtrl == encoderDimEnum.Encoder1D  ReferencedSubsystem=Encoder1D
  Encoder2D : Subsystem  VariantControl=encoderDimCtrl == encoderDimEnum.Encoder2D  ReferencedSubsystem=Encoder2D
  x : Outport  OutDataTypeStr=single
  y : Outport  Port=2  OutDataTypeStr=single

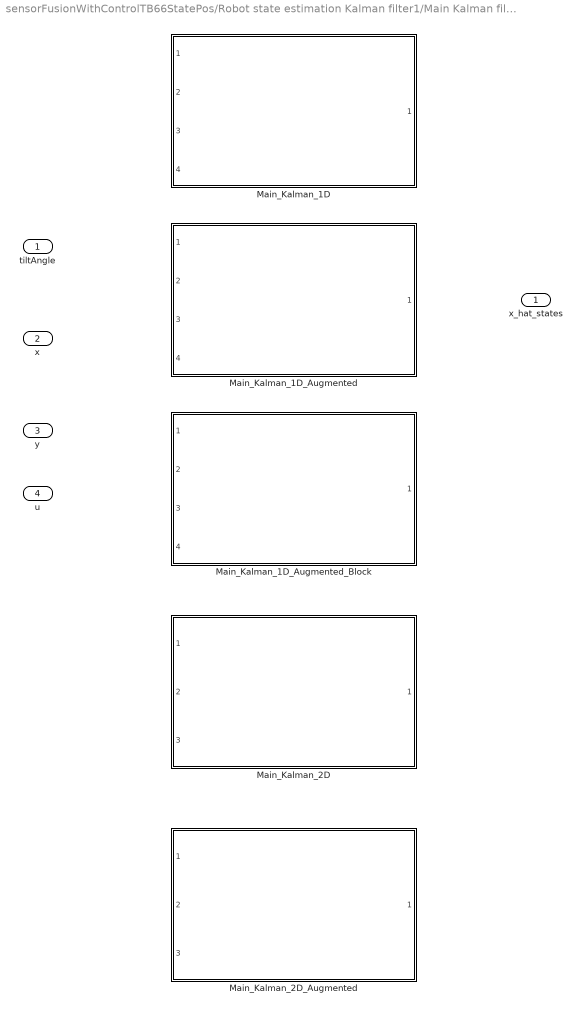
== system sensorFusionWithControlTB66StatePos/Robot state estimation Kalman filter1/Main Kalman filter ==
  tiltAngle : Inport  OutDataTypeStr=single
  x : Inport  Port=2  OutDataTypeStr=single
  y : Inport  Port=3  OutDataTypeStr=single
  u : Inport  Port=4  OutDataTypeStr=single
  Main_Kalman_1D : Subsystem  VariantControl=mainStateEstCtrl == mainStateEnum.Main_Kalman_1D  ReferencedSubsystem=Main_Kalman_1D
  Main_Kalman_1D_Augmented : Subsystem  VariantControl=mainStateEstCtrl == mainStateEnum.Main_Kalman_1D_Augmented  ReferencedSubsystem=Main_Kalman_1D_Augmented
  Main_Kalman_1D_Augmented_Block : Subsystem  VariantControl=mainStateEstCtrl == mainStateEnum.Main_Kalman_1D_Augmented_Block  ReferencedSubsystem=Main_Kalman_1D_Augmented_Block
  Main_Kalman_2D : Subsystem  VariantControl=mainStateEstCtrl == mainStateEnum.Main_Kalman_2D  ReferencedSubsystem=Main_Kalman_2D
  Main_Kalman_2D_Augmented : Subsystem  VariantControl=mainStateEstCtrl == mainStateEnum.Main_Kalman_2D_Augmented  ReferencedSubsystem=Main_Kalman_2D_Augmented
  x_hat_states : Outport  OutDataTypeStr=single
